simulink model "target_driver_2022_Ctrl_v_2_4_landing_2017a"  (R2017a)
settings: Solver=FixedStepDiscrete  StartTime=0.0  StopTime=13  FixedStep=0.0001  RelTol=1e-3  EnableMultiTasking=on
values from neighbouring files (symbols this model uses):
  a2_lb = -0.25    [target_driver_setup_2022_Ctrl_V_2_4.m]    (also in target_driver_setup_2022_Ctrl_V_2_4_christian.m)
  a2_openloop = -0    (= 0)    [target_driver_setup_2022_Ctrl_V_2_4.m]    (also in target_driver_setup_2022_Ctrl_V_2_4_christian.m)
  a2_ub = 0.25    [target_driver_setup_2022_Ctrl_V_2_4.m]    (also in target_driver_setup_2022_Ctrl_V_2_4_christian.m)
  adaptive_flag = 0    [target_driver_setup_2022_Ctrl_V_2_4.m]    (also in target_driver_setup_2022_Ctrl_V_2_4_christian.m)
  adaptive_gain = [gamma_adaptive, adaptive_roll_limit, adaptive_pitch_limit, adaptive_yaw_limit, c_2_adaptive, gamma_lateral_adaptive, adaptive_x_limit, adaptive_y_limit, adaptive_z_limit, c_1_adaptive]    [target_driver_setup_2022_Ctrl_V_2_4.m]    (also in target_driver_setup_2022_Ctrl_V_2_4_christian.m)
  adaptive_lateral_flag = 0    [target_driver_setup_2022_Ctrl_V_2_4.m]    (also in target_driver_setup_2022_Ctrl_V_2_4_christian.m)
  adaptive_pitch_init = 0    [target_driver_setup_2022_Ctrl_V_2_4.m]    (also in target_driver_setup_2022_Ctrl_V_2_4_christian.m)
  adaptive_pitch_limit = 0.1/(scale^2)    (= 1e-07)    [target_driver_setup_2022_Ctrl_V_2_4.m]    (also in target_driver_setup_2022_Ctrl_V_2_4_christian.m)
  adaptive_pitch_limit_low = -adaptive_pitch_limit    (= -1e-07)    [target_driver_setup_2022_Ctrl_V_2_4.m]    (also in target_driver_setup_2022_Ctrl_V_2_4_christian.m)
  adaptive_roll_init = 0    [target_driver_setup_2022_Ctrl_V_2_4.m]    (also in target_driver_setup_2022_Ctrl_V_2_4_christian.m)
  adaptive_roll_limit = 0.3/(scale^2)    (= 3e-07)    [target_driver_setup_2022_Ctrl_V_2_4.m]    (also in target_driver_setup_2022_Ctrl_V_2_4_christian.m)
  adaptive_roll_limit_low = -adaptive_roll_limit    (= -3e-07)    [target_driver_setup_2022_Ctrl_V_2_4.m]    (also in target_driver_setup_2022_Ctrl_V_2_4_christian.m)
  adaptive_x_init = 0    [target_driver_setup_2022_Ctrl_V_2_4.m]    (also in target_driver_setup_2022_Ctrl_V_2_4_christian.m)
  adaptive_x_limit = 0.15/(scale)    (= 0.00015)    [target_driver_setup_2022_Ctrl_V_2_4.m]    (also in target_driver_setup_2022_Ctrl_V_2_4_christian.m)
  adaptive_x_limit_low = -adaptive_x_limit    (= -0.00015)    [target_driver_setup_2022_Ctrl_V_2_4.m]    (also in target_driver_setup_2022_Ctrl_V_2_4_christian.m)
  adaptive_y_init = 0    [target_driver_setup_2022_Ctrl_V_2_4.m]    (also in target_driver_setup_2022_Ctrl_V_2_4_christian.m)
  adaptive_y_limit = 0.15/(scale)    (= 0.00015)    [target_driver_setup_2022_Ctrl_V_2_4.m]    (also in target_driver_setup_2022_Ctrl_V_2_4_christian.m)
  adaptive_y_limit_low = -adaptive_y_limit    (= -0.00015)    [target_driver_setup_2022_Ctrl_V_2_4.m]    (also in target_driver_setup_2022_Ctrl_V_2_4_christian.m)
  adaptive_yaw_init = 0    [target_driver_setup_2022_Ctrl_V_2_4.m]    (also in target_driver_setup_2022_Ctrl_V_2_4_christian.m)
  adaptive_yaw_limit = 0.035/(scale^2)    (= 3.5e-08)    [target_driver_setup_2022_Ctrl_V_2_4.m]    (also in target_driver_setup_2022_Ctrl_V_2_4_christian.m)
  adaptive_yaw_limit_low = -adaptive_yaw_limit    (= -3.5e-08)    [target_driver_setup_2022_Ctrl_V_2_4.m]    (also in target_driver_setup_2022_Ctrl_V_2_4_christian.m)
  adaptive_z_init = 0/scale    (= 0)    [target_driver_setup_2022_Ctrl_V_2_4.m]    (also in target_driver_setup_2022_Ctrl_V_2_4_christian.m)
  adaptive_z_limit = 0.20/(scale)    (= 0.0002)    [target_driver_setup_2022_Ctrl_V_2_4.m]    (also in target_driver_setup_2022_Ctrl_V_2_4_christian.m)
  adaptive_z_limit_low = -adaptive_z_limit/1    (= -0.0002)    [target_driver_setup_2022_Ctrl_V_2_4.m]    (also in target_driver_setup_2022_Ctrl_V_2_4_christian.m)
  att_s = 500    [target_driver_setup_2022_Ctrl_V_2_4.m]    (also in target_driver_setup_2022_Ctrl_V_2_4_christian.m)
  b_1_d_desired = [1,0,0]    [target_driver_setup_2022_Ctrl_V_2_4.m]    (also in target_driver_setup_2022_Ctrl_V_2_4_christian.m)
  closedloop_flag = 1    [target_driver_setup_2022_Ctrl_V_2_4.m]    (also in target_driver_setup_2022_Ctrl_V_2_4_christian.m)
  control_gain = [k_x,k_v, k_R, k_Omega, k_z, k_vz, k_Rx]    [target_driver_setup_2022_Ctrl_V_2_4.m]    (also in target_driver_setup_2022_Ctrl_V_2_4_christian.m)
  delay = delay-vicon_sample_cycle/2    [target_driver_setup_2022_Ctrl_V_2_4.m]    (also in target_driver_setup_2022_Ctrl_V_2_4_christian.m)
  drv_amp = 160    [target_driver_setup_2022_Ctrl_V_2_4.m]    (also in target_driver_setup_2022_Ctrl_V_2_4_christian.m)
  drv_bias = max_drv_bias    (= 300)    [target_driver_setup_2022_Ctrl_V_2_4.m]    (also in target_driver_setup_2022_Ctrl_V_2_4_christian.m)
  drv_pitch_left = 0    [target_driver_setup_2022_Ctrl_V_2_4.m]    (also in target_driver_setup_2022_Ctrl_V_2_4_christian.m)
  drv_pitch_right = 0    [target_driver_setup_2022_Ctrl_V_2_4.m]    (also in target_driver_setup_2022_Ctrl_V_2_4_christian.m)
  drv_roll = -2    [target_driver_setup_2022_Ctrl_V_2_4.m]    (also in target_driver_setup_2022_Ctrl_V_2_4_christian.m = 0)
  f_fin = f    (= 155)    [target_driver_setup_2022_Ctrl_V_2_4.m]    (also in target_driver_setup_2022_Ctrl_V_2_4_christian.m)
  f_int = f    (= 155)    [target_driver_setup_2022_Ctrl_V_2_4.m]    (also in target_driver_setup_2022_Ctrl_V_2_4_christian.m)
  g = 9.8    [target_driver_setup_2022_Ctrl_V_2_4.m]    (also in target_driver_setup_2022_Ctrl_V_2_4_christian.m)
  I_moment_vec = [Ixx, Iyy, Izz]    [target_driver_setup_2022_Ctrl_V_2_4.m]    (also in target_driver_setup_2022_Ctrl_V_2_4_christian.m)
  landing_flag = 0    [target_driver_setup_2022_Ctrl_V_2_4.m]    (also in target_driver_setup_2022_Ctrl_V_2_4_christian.m)
  landing_parameter = [start_delay+T,transition_rate, rising_time, falling_time, landing_rising_time, landing_z_decrease, landing_y_decrease, landing_x_decrease]    [target_driver_setup_2022_Ctrl_V_2_4.m]    (also in target_driver_setup_2022_Ctrl_V_2_4_christian.m = [start_delay+T, transition_rate, rising_time, falling_time, )
  low_bound = -8    [target_driver_setup_2022_Ctrl_V_2_4.m]    (also in target_driver_setup_2022_Ctrl_V_2_4_christian.m = -10)
  low_bound_eR = -0.8    [target_driver_setup_2022_Ctrl_V_2_4.m]    (also in target_driver_setup_2022_Ctrl_V_2_4_christian.m)
  low_bound_vx = -0.5    [target_driver_setup_2022_Ctrl_V_2_4.m]    (also in target_driver_setup_2022_Ctrl_V_2_4_christian.m)
  low_bound_vy = -0.5    [target_driver_setup_2022_Ctrl_V_2_4.m]    (also in target_driver_setup_2022_Ctrl_V_2_4_christian.m)
  low_bound_vz = -0.5    [target_driver_setup_2022_Ctrl_V_2_4.m]    (also in target_driver_setup_2022_Ctrl_V_2_4_christian.m)
  low_bound_x = -0.06    [target_driver_setup_2022_Ctrl_V_2_4.m]    (also in target_driver_setup_2022_Ctrl_V_2_4_christian.m)
  low_bound_y = -0.06    [target_driver_setup_2022_Ctrl_V_2_4.m]    (also in target_driver_setup_2022_Ctrl_V_2_4_christian.m)
  low_bound_z = -0.04    [target_driver_setup_2022_Ctrl_V_2_4.m]    (also in target_driver_setup_2022_Ctrl_V_2_4_christian.m)
  m = m+payload    (= 0.000124)    [target_driver_setup_2022_Ctrl_V_2_4.m]    (also in target_driver_setup_2022_Ctrl_V_2_4_christian.m = 0.000119)
  params_vec = [params_opt.delta_1, params_opt.delta_2, params_opt.delta_3, params_opt.gamma_1, params_opt.gamma_2, params_opt.gamma_3, params_opt.eta, params_opt.nu, params_opt.mu]'    [target_driver_setup_2022_Ctrl_V_2_4.m]    (also in target_driver_setup_2022_Ctrl_V_2_4_christian.m)
  phase = 0    [target_driver_setup_2022_Ctrl_V_2_4.m]    (also in target_driver_setup_2022_Ctrl_V_2_4_christian.m)
  r_desired = [default_x, default_y,z_desired]    [target_driver_setup_2022_Ctrl_V_2_4.m]    (also in target_driver_setup_2022_Ctrl_V_2_4_christian.m)
  roll_offset_angle = 0    [target_driver_setup_2022_Ctrl_V_2_4.m]    (also in target_driver_setup_2022_Ctrl_V_2_4_christian.m)
  running_time = start_delay+total_T    (= 8.5)    [target_driver_setup_2022_Ctrl_V_2_4.m]    (also in target_driver_setup_2022_Ctrl_V_2_4_christian.m = 8.4)
  running_time_control = start_delay_control+total_T+0.0    (= 8.6)    [target_driver_setup_2022_Ctrl_V_2_4.m]    (also in target_driver_setup_2022_Ctrl_V_2_4_christian.m = 8.5)
  start_delay = 2.0    (= 2)    [target_driver_setup_2022_Ctrl_V_2_4.m]    (also in target_driver_setup_2022_Ctrl_V_2_4_christian.m)
  start_delay_control = start_delay + ramp_delay    (= 2.1)    [target_driver_setup_2022_Ctrl_V_2_4.m]    (also in target_driver_setup_2022_Ctrl_V_2_4_christian.m)
  T = 0.5    [target_driver_setup_2022_Ctrl_V_2_4.m]    (also in target_driver_setup_2022_Ctrl_V_2_4_christian.m = 0.4)
  task_flag = 0    [target_driver_setup_2022_Ctrl_V_2_4.m]    (also in target_driver_setup_2022_Ctrl_V_2_4_christian.m)
  task_parameter = [radius_ref, frequency_ref, radius_ratio, lissajous_ratio, lissajous_delta, lissajous_amplitude_ratio,z_radius_ratio]    [target_driver_setup_2022_Ctrl_V_2_4.m]    (also in target_driver_setup_2022_Ctrl_V_2_4_christian.m)
  upp_bound = 8    [target_driver_setup_2022_Ctrl_V_2_4.m]    (also in target_driver_setup_2022_Ctrl_V_2_4_christian.m = 10)
  upp_bound_eR = 0.8    [target_driver_setup_2022_Ctrl_V_2_4.m]    (also in target_driver_setup_2022_Ctrl_V_2_4_christian.m)
  upp_bound_vx = 0.5    [target_driver_setup_2022_Ctrl_V_2_4.m]    (also in target_driver_setup_2022_Ctrl_V_2_4_christian.m)
  upp_bound_vy = 0.5    [target_driver_setup_2022_Ctrl_V_2_4.m]    (also in target_driver_setup_2022_Ctrl_V_2_4_christian.m)
  upp_bound_vz = 0.5    [target_driver_setup_2022_Ctrl_V_2_4.m]    (also in target_driver_setup_2022_Ctrl_V_2_4_christian.m)
  upp_bound_x = 0.06    [target_driver_setup_2022_Ctrl_V_2_4.m]    (also in target_driver_setup_2022_Ctrl_V_2_4_christian.m)
  upp_bound_y = 0.06    [target_driver_setup_2022_Ctrl_V_2_4.m]    (also in target_driver_setup_2022_Ctrl_V_2_4_christian.m)
  upp_bound_z = 0.04    [target_driver_setup_2022_Ctrl_V_2_4.m]    (also in target_driver_setup_2022_Ctrl_V_2_4_christian.m)
undefined symbols (not defined in the file or in its folder): A, Com1, DiscIntNeverNeededParam, left_mapping, left_mapping_F_to_Phi, lp_den, lp_num, none, right_mapping, right_mapping_F_to_Phi, vlp_den, vlp_num
libraries: simulink x25, xpcnilib x2, xpcseriallib x2, xpcutilitieslib x1
(part 4 of 4)

== system target_driver_2022_Ctrl_v_2_4_landing_2017a/signal generator a1/Drive_Signal/FlattenedSine1/AveragedAmp_filtered ==
  note: To avoid having signal "jump",
      | we want SMOOTH transitions
      | in frequency (i.e., a weighted sum
      | of current freq and freq some delta t ago)
  note: time constant 0.002sec
      | for 10kHz samping
  In1 : Inport
  Discrete Transfer Fcn : DiscreteTransferFcn  Numerator=[0.05]  Denominator=[1 -.95]
  Out1 : Outport
  wires:
  In1/1 -> Discrete Transfer Fcn/1
  Discrete Transfer Fcn/1 -> Out1/1

== system target_driver_2022_Ctrl_v_2_4_landing_2017a/signal generator a1/Drive_Signal1/FlattenedSine1/Amplitude Correction ==
  y : Inport
  a2 : Inport  Port=2
  Abs : Abs
  Constant : Constant  Value=1.2
  Constant1 : Constant  Value=1.1
  Divide : Product  Inputs=*/
  Product1 : Product
  Sqrt : Sqrt  SaturateOnIntegerOverflow=on
  Subtract : Sum  Inputs=+-
  y_new : Outport
  wires:
  Constant/1 -> Subtract/1
  Subtract/1 -> Sqrt/1
  Abs/1 -> Subtract/2
  a2/1 -> Abs/1
  y/1 -> Product1/1
  Product1/1 -> y_new/1
  Divide/1 -> Product1/2
  Constant1/1 -> Divide/2
  Sqrt/1 -> Divide/1

== system target_driver_2022_Ctrl_v_2_4_landing_2017a/signal generator a1/Drive_Signal1/FlattenedSine1/AveragedAmp_filtered ==
  note: To avoid having signal "jump",
      | we want SMOOTH transitions
      | in frequency (i.e., a weighted sum
      | of current freq and freq some delta t ago)
  note: time constant 0.002sec
      | for 10kHz samping
  In1 : Inport
  Discrete Transfer Fcn : DiscreteTransferFcn  Numerator=[0.05]  Denominator=[1 -.95]
  Out1 : Outport
  wires:
  In1/1 -> Discrete Transfer Fcn/1
  Discrete Transfer Fcn/1 -> Out1/1

== system target_driver_2022_Ctrl_v_2_4_landing_2017a/signal generator a2/Drive_Signal/FlattenedSine1/Amplitude Correction ==
  y : Inport
  a2 : Inport  Port=2
  Abs : Abs
  Constant : Constant  Value=1.2
  Constant1 : Constant  Value=1.1
  Divide : Product  Inputs=*/
  Product1 : Product
  Sqrt : Sqrt  SaturateOnIntegerOverflow=on
  Subtract : Sum  Inputs=+-
  y_new : Outport
  wires:
  Constant/1 -> Subtract/1
  Subtract/1 -> Sqrt/1
  Abs/1 -> Subtract/2
  a2/1 -> Abs/1
  y/1 -> Product1/1
  Product1/1 -> y_new/1
  Divide/1 -> Product1/2
  Constant1/1 -> Divide/2
  Sqrt/1 -> Divide/1

== system target_driver_2022_Ctrl_v_2_4_landing_2017a/signal generator a2/Drive_Signal1/FlattenedSine1/Amplitude Correction ==
  y : Inport
  a2 : Inport  Port=2
  Abs : Abs
  Constant : Constant  Value=1.2
  Constant1 : Constant  Value=1.1
  Divide : Product  Inputs=*/
  Product1 : Product
  Sqrt : Sqrt  SaturateOnIntegerOverflow=on
  Subtract : Sum  Inputs=+-
  y_new : Outport
  wires:
  Constant/1 -> Subtract/1
  Subtract/1 -> Sqrt/1
  Abs/1 -> Subtract/2
  a2/1 -> Abs/1
  y/1 -> Product1/1
  Product1/1 -> y_new/1
  Divide/1 -> Product1/2
  Constant1/1 -> Divide/2
  Sqrt/1 -> Divide/1

== matlab function target_driver_2022_Ctrl_v_2_4_landing_2017a/Observer for averaged system/Attitude Observer/Geometric Averaging Rotation Matix/Raw quaternion ==
  data: R input; quat output
function quat = fcn(R)
Rot = zeros(3,3);
Rot = [R(1), R(2), R(3); R(4), R(5), R(6); R(7), R(8), R(9); ];
quat = rotm2quat(Rot)';

== matlab function target_driver_2022_Ctrl_v_2_4_landing_2017a/Open_Closed_loop_selection/MATLAB Function ==
  data: time input; freq output; f_int parameter; f_fin parameter; T parameter
function freq = fcn(time, f_int, f_fin, T)
%#codegen

freq = f_int;
buffer_t = 0.0; %3.0
rel_time = time-buffer_t;
if rel_time > 0
    freq = f_int + (f_fin-f_int) * (rel_time/T);
end

if freq > f_fin
    freq = f_fin;
end

== matlab function target_driver_2022_Ctrl_v_2_4_landing_2017a/Geometric Controller/Geometric Controller ==
  data: thrust_desired output; R_cur input; R_desired input; omega input; roll_torque_desired output; omega_desired input; omega_d_dot input; x_d_ddot input; e_x input; e_v input; e_R input; e_Omega input; control_gain input; I_moment_vec input; pitch_torque_desired output; m input; g input; yaw_torque_desired output; adaptive_roll input; adaptive_pitch input; adaptive_yaw input; adaptive_x input; adaptive_y input; adaptive_z input
function [thrust_desired, roll_torque_desired, pitch_torque_desired, yaw_torque_desired] = fcn(R_cur,R_desired, omega, omega_desired, omega_d_dot,x_d_ddot,e_x,e_v,e_R,e_Omega,control_gain,I_moment_vec, m, g, adaptive_roll,adaptive_pitch, adaptive_yaw, adaptive_x,adaptive_y, adaptive_z)
% 
Rot_cur = [R_cur(1), R_cur(2), R_cur(3); R_cur(4), R_cur(5), R_cur(6); R_cur(7), R_cur(8), R_cur(9)];
Rot_desired = [R_desired(1), R_desired(2), R_desired(3); R_desired(4), R_desired(5), R_desired(6); R_desired(7), R_desired(8), R_desired(9)];

k_x=control_gain(1);
k_v=control_gain(2);
k_R=control_gain(3);
k_Omega=control_gain(4);
k_z=control_gain(5);
k_vz=control_gain(6);
k_Rx=control_gain(7);

e_3 = [0,0,1]';
I_moment = zeros(3,3);
I_moment(1,1) = I_moment_vec(1);
I_moment(2,2) = I_moment_vec(2);
I_moment(3,3) = I_moment_vec(3);

w_hat=zeros(3,3);

w_hat(1,2) = -omega(3);
w_hat(2,1) = omega(3);
w_hat(1,3) = omega(2);
w_hat(3,1) = -omega(2);
w_hat(2,3) = -omega(1);
w_hat(3,2) = omega(1);

K_X = [k_x;k_x;k_z];
K_V = [k_v;k_v;k_vz];

% Different attitude gain
K_R = [k_Rx;k_R;k_R];

% Geoemtri Controller in SE(3)

M = -K_R.*e_R - k_Omega*e_Omega + w_hat*I_moment*omega - ...
                I_moment*(w_hat*Rot_cur'*Rot_desired*omega_desired - Rot_cur'*Rot_desired*omega_d_dot);

% Adaptive torques

roll_torque_desired = M(1)-adaptive_roll;
pitch_torque_desired = M(2)-adaptive_pitch;
yaw_torque_desired = M(3)/6-adaptive_yaw;

% Geometric Lateral control in SE(3)
adaptive_lateral = [adaptive_x; adaptive_y; adaptive_z];

f = (-K_X.*e_x - K_V.*e_v -adaptive_lateral + m*g*e_3 + m*x_d_ddot)'*Rot_cur*e_3;

thrust_desired = f;




if thrust_desired >= 1.6e-3
	thrust_desired= 1.6e-3;
elseif thrust_desired <=0.5e-3
	thrust_desired=0.5e-3;
end

if roll_torque_desired >= 0.5e-6
		roll_torque_desired=0.5e-6;
elseif roll_torque_desired <= -0.6e-6
		roll_torque_desired=-0.6e-6;
end

if pitch_torque_desired >= 0.2e-6
		pitch_torque_desired=0.2e-6;
elseif pitch_torque_desired <= -0.2e-6
		pitch_torque_desired=-0.2e-6;
end

% if yaw_torque_desired >= 0.2e-7
% 		pitch_torque_desired=0.2e-7;
% elseif yaw_torque_desired <= -0.2e-7
% 		yaw_torque_desired=-0.2e-7;
% end
if yaw_torque_desired >= 0.9e-7
	yaw_torque_desired = 0.9e-7;
elseif yaw_torque_desired <= -1.0e-7
	yaw_torque_desired = -1.0e-7;
end

end

== matlab function target_driver_2022_Ctrl_v_2_4_landing_2017a/Open_Closed_loop_selection/MATLAB Function4 ==
  data: openloop_control input; closedloop_control input; drv_amp_final output; closedloop_flag input; drv_pch_final_left output; drv_pch_final_right output; drv_roll_final output; a2_final output
function [drv_amp_final, drv_pch_final_left,drv_pch_final_right, drv_roll_final, a2_final] = fcn(openloop_control, closedloop_control, closedloop_flag)

if closedloop_flag==1
    drv_amp_final =closedloop_control(1);
    drv_pch_final_left =closedloop_control(2);
		drv_pch_final_right =closedloop_control(3);
    drv_roll_final=closedloop_control(4);
		a2_final=closedloop_control(5);
else
    drv_amp_final =openloop_control(1);
    drv_pch_final_left =openloop_control(2);
		drv_pch_final_right =openloop_control(3);
    drv_roll_final=openloop_control(4);
		a2_final=openloop_control(5);
		
end

== matlab function target_driver_2022_Ctrl_v_2_4_landing_2017a/Observer for averaged system/Position Observer/Averaging position & velocity  ==
  data: r_prev input; r_prev2 input; r_prev3 input; r_cur input; update input; count input; rout_prev input; rout output; vout_prev input; vout output
function [rout, vout] = fcn(r_prev,r_prev2,r_prev3,r_cur,update, count,rout_prev,vout_prev)
%#codegen

rout = zeros(3,1);
vout = zeros(3,1);
if update>0
   rout=rout_prev; 
   vout=vout_prev;
else

    % 1 cycle average
    n= 4;
    
    rout = (r_prev+r_prev2+r_prev3+r_cur)/n;
    vout = (rout-rout_prev)*10000/(count+1);
    
  
end

end

== matlab function target_driver_2022_Ctrl_v_2_4_landing_2017a/Geometric Controller/lateral adaptive/Adaptive Control ==
  data: current_adaptive_x input; current_adaptive_y input; current_adaptive_z input; der_adaptive_torque_x output; e_x input; e_v input; adaptive_gain_limit input; der_adaptive_torque_y output; der_adaptive_torque_z output
function [der_adaptive_torque_x, der_adaptive_torque_y, der_adaptive_torque_z] = fcn(current_adaptive_x,current_adaptive_y,current_adaptive_z, e_x,e_v,adaptive_gain_limit)


% Current state of adaptation
adaptive_torque_x=current_adaptive_x;
adaptive_torque_y=current_adaptive_y;
adaptive_torque_z=current_adaptive_z;

% Adaptive control parameters
gamma_lateral_adaptive = adaptive_gain_limit(6);
adaptvie_x_limit = adaptive_gain_limit(7);
adaptvie_y_limit = adaptive_gain_limit(8);
adaptvie_z_limit = adaptive_gain_limit(9);
c_1 = adaptive_gain_limit(10);

% Flag indicating the limit
adaptive_flag_x = adaptive_torque_x*(e_v(1)+c_1*e_x(1));
adaptive_flag_y = adaptive_torque_y*(e_v(2)+c_1*e_x(2));
adaptive_flag_z = adaptive_torque_z*(e_v(3)+c_1*e_x(3));

% size(adaptive_flag_x)

% derivative for desired adaptation
der_adaptive = gamma_lateral_adaptive*(e_v+c_1*e_x);

% epsillon=1e-15;


if (adaptive_flag_x<=0 && abs(adaptive_torque_x)==adaptvie_x_limit) || abs(adaptive_torque_x)<adaptvie_x_limit
	
	der_adaptive_torque_x=der_adaptive(1);
else
	der_adaptive_torque_x = 0;
end

if (adaptive_flag_y<=0 && abs(adaptive_torque_y)==adaptvie_y_limit) || abs(adaptive_torque_y)<adaptvie_y_limit
	
	der_adaptive_torque_y=der_adaptive(2);
else
	der_adaptive_torque_y = 0;
	
end

if (adaptive_flag_z<=0 && abs(adaptive_torque_z)==adaptvie_z_limit)|| abs(adaptive_torque_z)<adaptvie_z_limit
	
	der_adaptive_torque_z=der_adaptive(3);
else
	der_adaptive_torque_z = 0;
	
end


end

== matlab function target_driver_2022_Ctrl_v_2_4_landing_2017a/Observer for averaged system/Euler derivative & filtered angular velocity /Angular velocity ==
  data: R input; Rdot input; w output; Frob_error output
function [w,Frob_error] = fcn(R,Rdot)
%#codegen
Rot = [R(1), R(2), R(3); R(4), R(5), R(6); R(7), R(8), R(9); ];
dRot = [Rdot(1), Rdot(2), Rdot(3); Rdot(4), Rdot(5), Rdot(6); Rdot(7), Rdot(8), Rdot(9); ];

A = Rot'*dRot;
w_hat = 1/2*(A-A');
w=zeros(3,1);
w(1) = w_hat(3,2);
w(2) = w_hat(1,3);
w(3) = w_hat(2,1);
% wz = w(3);
Frob_error=trace((A+A')*(A+A'));

== matlab function target_driver_2022_Ctrl_v_2_4_landing_2017a/Vicon Post Processing/Vicon Validity check/MATLAB Function3 ==
  data: R_prev input; y output; R_cur input
function y = fcn(R_prev,R_cur)
Rot_cur = [R_cur(1), R_cur(2), R_cur(3); R_cur(4), R_cur(5), R_cur(6); R_cur(7), R_cur(8), R_cur(9)];
Rot_prev = [R_prev(1), R_prev(2), R_prev(3); R_prev(4), R_prev(5), R_prev(6); R_prev(7), R_prev(8), R_prev(9)];

A=Rot_cur'*Rot_prev;
epsilonn = 1e-18;

if trace((A-eye(3))'*(A-eye(3)))<epsilonn
   y=0; 
else
    y=1;
end

== matlab function target_driver_2022_Ctrl_v_2_4_landing_2017a/Vicon correction ==
  data: x_cur input; x_corrected_vec output; roll_offset_angle input
function x_corrected_vec = fcn(x_cur,roll_offset_angle)

x_cur_vec = [x_cur(1); x_cur(2); x_cur(3)];
Rot_correction = [1, 0, 0; ...
									0, cos(roll_offset_angle), -sin(roll_offset_angle);...
									0, sin(roll_offset_angle), cos(roll_offset_angle)];
x_corrected_vec = Rot_correction*x_cur_vec;

end

== matlab function target_driver_2022_Ctrl_v_2_4_landing_2017a/Desired attitude and normalized error/saturated normalized error observation/Saturated angular velocity eOmega /Compute attitude error eR ==
  data: y output; R_cur input; R_desired input; omega input; omega_desired input
function y  = fcn(R_cur,R_desired,omega, omega_desired)

Rot_cur = [R_cur(1), R_cur(2), R_cur(3); R_cur(4), R_cur(5), R_cur(6); R_cur(7), R_cur(8), R_cur(9)];
Rot_desired = [R_desired(1), R_desired(2), R_desired(3); R_desired(4), R_desired(5), R_desired(6); R_desired(7), R_desired(8), R_desired(9)];
eOmega=zeros(3,1);
eOmega = omega - Rot_cur'*Rot_desired*omega_desired;

y = eOmega;

end

== matlab function target_driver_2022_Ctrl_v_2_4_landing_2017a/Observer for averaged system/Attitude Observer/Geometric Averaging Rotation Matix/Geometric Averaging Rotation M/Geometric Average  ==
  data: R_prev input; R_prev2 input; R_prev3 input; R_prev4 input; R_prev5 input; R_prev6 input; Rout output; R_cur input; update input; Rout_prev input
function Rout = fcn(R_prev,R_prev2,R_prev3,R_prev4,R_prev5,R_prev6,R_cur,update,Rout_prev)
%#codegen
Rot_cur = [R_cur(1), R_cur(2), R_cur(3); R_cur(4), R_cur(5), R_cur(6); R_cur(7), R_cur(8), R_cur(9)];
Rot_prev = [R_prev(1), R_prev(2), R_prev(3); R_prev(4), R_prev(5), R_prev(6); R_prev(7), R_prev(8), R_prev(9)];
Rot_prev2 = [R_prev2(1), R_prev2(2), R_prev2(3); R_prev2(4), R_prev2(5), R_prev2(6); R_prev2(7), R_prev2(8), R_prev2(9)];
Rot_prev3 = [R_prev3(1), R_prev3(2), R_prev3(3); R_prev3(4), R_prev3(5), R_prev3(6); R_prev3(7), R_prev3(8), R_prev3(9)];
Rot_prev4 = [R_prev4(1), R_prev4(2), R_prev4(3); R_prev4(4), R_prev4(5), R_prev4(6); R_prev4(7), R_prev4(8), R_prev4(9)];
Rot_prev5 = [R_prev5(1), R_prev5(2), R_prev5(3); R_prev5(4), R_prev5(5), R_prev5(6); R_prev5(7), R_prev5(8), R_prev5(9)];
Rot_prev6 = [R_prev6(1), R_prev6(2), R_prev6(3); R_prev6(4), R_prev6(5), R_prev6(6); R_prev6(7), R_prev6(8), R_prev6(9)];

Rout = zeros(9,1);
if update>0
   Rout=Rout_prev; 
else
% % 1 cycle average
%     n= 3;
%     
%     w_R0 = exp_map(Rot_cur);
%     w_R1 = exp_map(Rot_prev);
%     w_R2 = exp_map(Rot_prev2);
%     
%     
%     if sign(w_R2'*w_R0)<0
%         w_R0=-w_R0;
%     end
%     if sign(w_R2'*w_R1)<0
%         w_R1=-w_R1;
%     end
%    
%     
%     meanR0=frac_rot(w_R0,n);
%     meanR1=frac_rot(w_R1,n);
%     meanR2=frac_rot(w_R2,n);
%    
%     mean_R = meanR2*meanR1*meanR0;

% 1 cycle average
    n= 4;
    
    w_R0 = exp_map(Rot_cur);
    w_R1 = exp_map(Rot_prev);
    w_R2 = exp_map(Rot_prev2);
    w_R3 = exp_map(Rot_prev3);
    
    
    if sign(w_R3'*w_R0)<0
        w_R0=-w_R0;
    end
    if sign(w_R3'*w_R1)<0
        w_R1=-w_R1;
    end
    if sign(w_R3'*w_R2)<0
        w_R2=-w_R2;
    end
    
    meanR0=frac_rot(w_R0,n);
    meanR1=frac_rot(w_R1,n);
    meanR2=frac_rot(w_R2,n);
    meanR3=frac_rot(w_R3,n);

    mean_R = meanR3*meanR2*meanR1*meanR0;

% % 2 cycle average
%     n=7;
%     w_R0 = exp_map(Rot_cur);
%     w_R1 = exp_map(Rot_prev);
%     w_R2 = exp_map(Rot_prev2);
%     w_R3 = exp_map(Rot_prev3);
%     w_R4 = exp_map(Rot_prev4);
%     w_R5 = exp_map(Rot_prev5);
%     w_R6 = exp_map(Rot_prev6);
%     
%     if sign(w_R6'*w_R0)<0
%         w_R0=-w_R0;
%     end
%     if sign(w_R6'*w_R1)<0
%         w_R1=-w_R1;
%     end
%     if sign(w_R6'*w_R2)<0
%         w_R2=-w_R2;
%     end
%     if sign(w_R6'*w_R3)<0
%         w_R3=-w_R3;
%     end
%     if sign(w_R6'*w_R4)<0
%         w_R4=-w_R4;
%     end
%     if sign(w_R5'*w_R5)<0
%         w_R5=-w_R5;
%     end
%     meanR0=frac_rot(w_R0,n); 
%     meanR1=frac_rot(w_R1,n);
%     meanR2=frac_rot(w_R2,n);
%     meanR3=frac_rot(w_R3,n);
%     meanR4=frac_rot(w_R4,n);
%     meanR5=frac_rot(w_R5,n);
%     meanR6=frac_rot(w_R6,n);
% 
% %     mean_R = meanR3*meanR2*meanR1*meanR0;
%     mean_R = meanR6*meanR5*meanR4*meanR3*meanR2*meanR1*meanR0;
    
    Rout = [mean_R(1,1); mean_R(1,2); mean_R(1,3); mean_R(2,1); mean_R(2,2); mean_R(2,3); mean_R(3,1); mean_R(3,2); mean_R(3,3)]; 
end

end

function w = exp_map(R)

tr_R_diff = trace(R);
% isreal(tr_R_diff)
if abs((tr_R_diff-1)/2)<=1
    theta = acos((tr_R_diff-1)/2);
else
    theta=acos((tr_R_diff-1)/2/abs((tr_R_diff-1)/2));
end
if theta==0
    w= [0;0;0];
else
    w = theta/(2*sin(theta))*[R(3,2)-R(2,3); R(1,3) - R(3,1); R(2,1)-R(1,2)];
end
end

function fractional_rot = frac_rot(w,n)

w_hat = zeros(3,3);
w_hat = [0,-w(3),w(2);...
          w(3),0,-w(1);...
          -w(2), w(1), 0]/n;
fractional_rot = expm(w_hat);
end
% mean_R = R_prev_prev^(1/3)*R_prev^(1/3)*R_cur^(1/3);

% R is 1x9

== matlab function target_driver_2022_Ctrl_v_2_4_landing_2017a/Observer for averaged system/Attitude Observer/Geometric Averaging Rotation Matix/Averaged quaternion ==
  data: R input; quat output
function quat = fcn(R)
Rot = zeros(3,3);
Rot = [R(1), R(2), R(3); R(4), R(5), R(6); R(7), R(8), R(9); ];
quat = rotm2quat(Rot)';

== matlab function target_driver_2022_Ctrl_v_2_4_landing_2017a/Observer for averaged system/Attitude Observer/Geometric derivative in SO(3)/First order geometric derivative in SO(3)  ==
  data: R_prev input; omega output; R_cur input; omega_prev input; update input; count input
function omega  = fcn(R_prev, R_cur, omega_prev, update, count)

Rot_cur = [R_cur(1), R_cur(2), R_cur(3); R_cur(4), R_cur(5), R_cur(6); R_cur(7), R_cur(8), R_cur(9)];
Rot_prev = [R_prev(1), R_prev(2), R_prev(3); R_prev(4), R_prev(5), R_prev(6); R_prev(7), R_prev(8), R_prev(9)];

R_diff = Rot_prev'*Rot_cur;

tr_R_diff = trace(R_diff);
omega = zeros(3,1);
if update>0
   omega=omega_prev; 
else
    
% isreal(tr_R_diff)
if abs((tr_R_diff-1)/2)<=1
    theta = acos((tr_R_diff-1)/2);
else
    theta=acos((tr_R_diff-1)/2/abs((tr_R_diff-1)/2));
end

% To avoid NaN for omega
if theta<1e-10
	omega = omega_prev;
else
	w = 1/(2*sin(theta))*[R_diff(3,2)-R_diff(2,3); R_diff(1,3) - R_diff(3,1); R_diff(2,1)-R_diff(1,2)];

	omega = w*theta*10000/(count+1);
end   

end
% 
% if theta==0 %update~=0 
%     y = y_prev;
% else
%      w = 1/(2*sin(theta))*[R_diff(3,2)-R_diff(2,3); R_diff(1,3) - R_diff(3,1); R_diff(2,1)-R_diff(1,2)];
%      y = w*theta*10000/20;
% end

== matlab function target_driver_2022_Ctrl_v_2_4_landing_2017a/Phantom1/start at three ==
  data: time input; trigger output
function trigger = fcn(time)
%#codegen
trigger = 0;
if time > 0
   trigger = 1; 
end
if time > 0.1
   trigger = 0; 
end

== matlab function target_driver_2022_Ctrl_v_2_4_landing_2017a/Desired attitude and normalized error/saturated normalized error observation/Saturated normalized eR/Compute attitude error eR ==
  data: y output; R_cur input; R_desired input
function y  = fcn(R_cur,R_desired)

Rot_cur = [R_cur(1), R_cur(2), R_cur(3); R_cur(4), R_cur(5), R_cur(6); R_cur(7), R_cur(8), R_cur(9)];
Rot_desired = [R_desired(1), R_desired(2), R_desired(3); R_desired(4), R_desired(5), R_desired(6); R_desired(7), R_desired(8), R_desired(9)];
eR_so3=zeros(3,3);
eR_so3 = 1/2*(Rot_desired.'*Rot_cur-Rot_cur.'*Rot_desired);

eR = zeros(3,1);
eR(1) = eR_so3(3,2);
eR(2) = eR_so3(1,3);
eR(3) = eR_so3(2,1);

y = eR;

end

== matlab function target_driver_2022_Ctrl_v_2_4_landing_2017a/Force_to_Voltage1/Desired_Force_to_Voltage ==
  data: Thrust_desired input; drv_amp output; Roll_torque_desired input; Pitch_torque_desired input; Yaw_torque_desired input; drv_roll output; drv_pitch_left output; drv_pitch_right output; a2_coeff output; params_vec input
function [drv_amp, drv_roll, drv_pitch_left, drv_pitch_right, a2_coeff] =    fcn(Thrust_desired, Roll_torque_desired, Pitch_torque_desired, Yaw_torque_desired, params_vec)

% global params_opt

delta_1 = params_vec(1);
delta_2 = params_vec(2);
delta_3 = params_vec(3);
gamma_1 = params_vec(4);
gamma_2 = params_vec(5);
gamma_3 = params_vec(6);
eta = params_vec(7);
nu = params_vec(8);
mu = params_vec(9);


% Initializing for averaging filter at the end to prevent InF
if Thrust_desired==0    
    u4 = 0;
else
    u4 = Pitch_torque_desired/(Thrust_desired*delta_3*gamma_2)-nu;
end


% u3 calculation when tau approaches to zero
if abs(Yaw_torque_desired)<1e-12
    
   u3 = -mu;
else
    % Bounds for the mapping to produce real solution
    lb =(Thrust_desired/2)*(gamma_2*gamma_3*delta_2*mu/delta_1-sqrt((gamma_2*gamma_3*delta_2*Thrust_desired*mu/delta_1)^2+gamma_2*gamma_3));
    ub =(Thrust_desired/2)*(gamma_2*gamma_3*delta_2*mu/delta_1+sqrt((gamma_2*gamma_3*delta_2*Thrust_desired*mu/delta_1)^2+gamma_2*gamma_3));
   
   if Yaw_torque_desired>=ub
       Yaw_torque_desired = ub;
   elseif Yaw_torque_desired<=lb
       Yaw_torque_desired = lb; 
   end
       
   u3 = delta_1*(gamma_2*gamma_3*Thrust_desired-sqrt((gamma_2*gamma_3*Thrust_desired)^2-4*Yaw_torque_desired*(Yaw_torque_desired-gamma_2*gamma_3*delta_2*Thrust_desired*mu/delta_1)))/(2*delta_2*Yaw_torque_desired);

end

D = delta_1^2+delta_2^2*u3^2;
u1 = (gamma_2*Thrust_desired+Roll_torque_desired)/(2*gamma_1*gamma_2*D*eta);
u2 = (gamma_2*Thrust_desired-Roll_torque_desired)/(2*gamma_1*gamma_2*D);

vleft_p2p = sqrt(u1)*2;
vright_p2p = sqrt(u2)*2;
vleft_pitch = u4;
vright_pitch = u4;


drv_amp = abs((vleft_p2p-vright_p2p))/2+min(vleft_p2p,vright_p2p); % p2p
drv_roll = (vleft_p2p-vright_p2p)/4; % Amplitude
drv_pitch_left = vleft_pitch;
drv_pitch_right = vright_pitch;
a2_coeff = u3;

end

== matlab function target_driver_2022_Ctrl_v_2_4_landing_2017a/Desired attitude and normalized error/Desired_Attitude  ==
  data: R_cur input; R_d_prev input; R_d_vec output; e_x input; e_v input; x_d_ddot input; b_1_d input; control_gain input; m input; g input; update input; adaptive_lateral_control input
function R_d_vec = fcn(R_cur,R_d_prev, e_x,e_v,x_d_ddot, b_1_d, control_gain, m, g, update, adaptive_lateral_control)

R_d_vec = zeros(9,1);
data = 0;
if update>0
   R_d_vec=R_d_prev; 
	 
else
    
    k_x = control_gain(1);
    k_v = control_gain(2);
		k_z = control_gain(5);
		k_vz = control_gain(6);
		
		K_X = [k_x;k_x;k_z];
		K_V = [k_v;k_v;k_vz];

    e_3 = [0 0 1]';
%     e_1 = [1 0 0]';
		
    Rot_cur = [R_cur(1), R_cur(2), R_cur(3); R_cur(4), R_cur(5), R_cur(6); R_cur(7), R_cur(8), R_cur(9)];
		
% 		% Current heading control
%     b_1_d = Rot_cur*e_1;
% 		
% 		% Desired constant heading 
% 		b_1_d = [0 1 0]'; % e_1;
		
% Heading selection
    b_1_d = b_1_d/norm(b_1_d);

% Adaptive lateral control direction
adaptive_lateral = [adaptive_lateral_control(1); adaptive_lateral_control(2); adaptive_lateral_control(3)];
		

    b_3_d = (-K_X.*e_x - K_V.*e_v -adaptive_lateral + m*g*e_3 + m*x_d_ddot) / ...
            norm(-K_X.*e_x - K_V.*e_v -adaptive_lateral + m*g*e_3 + m*x_d_ddot);
    b_2_d = cross(b_3_d,b_1_d) / norm(cross(b_3_d,b_1_d));
		
% 		data = norm(b_2_d);
		
    % Desired rotation matrix
    R_d = [cross(b_2_d,b_3_d) b_2_d b_3_d];

    R_d_vec = [R_d(1,1); R_d(1,2); R_d(1,3); R_d(2,1); R_d(2,2); R_d(2,3); R_d(3,1); R_d(3,2); R_d(3,3)];

end



end

== matlab function target_driver_2022_Ctrl_v_2_4_landing_2017a/Force_to_Voltage1/Force to Trajectory  ==
  data: Thrust_desired input; Phi_left_p2p_desired output; Roll_torque_desired input; Pitch_torque_desired input; left_mapping_F_to_Phi input; right_mapping_F_to_Phi input; A input; Phi_right_p2p_desired output; Phi_pitch_desired output
function [Phi_left_p2p_desired, Phi_right_p2p_desired, Phi_pitch_desired] = fcn(Thrust_desired, Roll_torque_desired, Pitch_torque_desired, left_mapping_F_to_Phi, right_mapping_F_to_Phi, A)

delta_opt_L = left_mapping_F_to_Phi(1);
gamma_opt_L = left_mapping_F_to_Phi(2);
phi_opt_L = left_mapping_F_to_Phi(3);
phi_opt_offset_L = left_mapping_F_to_Phi(4);

delta_opt_R = right_mapping_F_to_Phi(1);
gamma_opt_R = right_mapping_F_to_Phi(2);
phi_opt_R = right_mapping_F_to_Phi(3);
phi_opt_offset_R = right_mapping_F_to_Phi(4);

T_thrust_roll = A*[ delta_opt_L              ,               delta_opt_R;...
                    delta_opt_L*gamma_opt_L  , - delta_opt_R*gamma_opt_R];
T_pitch_thrust = A*[delta_opt_L*gamma_opt_L  , delta_opt_R*gamma_opt_R].*[phi_opt_L, phi_opt_R];
T_pitch_offset = A*[delta_opt_L*gamma_opt_L  , delta_opt_R*gamma_opt_R].*[phi_opt_offset_L, phi_opt_offset_R];

Thrust_roll = [Thrust_desired; Roll_torque_desired];
u1_u2_desired = (T_thrust_roll)\Thrust_roll;

if (T_pitch_thrust*u1_u2_desired)==0
	Phi_pitch_desired = 0;
else
	Phi_pitch_desired = (Pitch_torque_desired-T_pitch_offset*u1_u2_desired)/(T_pitch_thrust*u1_u2_desired);
end

Phi_left_p2p_desired = sqrt(u1_u2_desired(1));
Phi_right_p2p_desired = sqrt(u1_u2_desired(2));

== matlab function target_driver_2022_Ctrl_v_2_4_landing_2017a/Desired attitude and normalized error/Geometric derivative for Rd in SO(3)/First order geometric derivative in SO(3)  ==
  data: R_prev input; omega_d output; R_cur input; omega_d_prev input; update input; count input
function omega_d   = fcn(R_prev, R_cur, omega_d_prev, update, count)

Rot_cur = [R_cur(1), R_cur(2), R_cur(3); R_cur(4), R_cur(5), R_cur(6); R_cur(7), R_cur(8), R_cur(9)];
Rot_prev = [R_prev(1), R_prev(2), R_prev(3); R_prev(4), R_prev(5), R_prev(6); R_prev(7), R_prev(8), R_prev(9)];

R_diff = Rot_prev'*Rot_cur;

tr_R_diff = trace(R_diff);
omega_d = zeros(3,1);
% omega_d_dot = zeros(3,1);

if update>0
   omega_d=omega_d_prev; 
%    omega_d_dot = omega_d_dot_prev;
else
    
% isreal(tr_R_diff)
if abs((tr_R_diff-1)/2)<=1
    theta = acos((tr_R_diff-1)/2);
else
    theta=acos((tr_R_diff-1)/2/abs((tr_R_diff-1)/2));
end

if theta==0
	theta=1e-14;
end

   w = 1/(2*sin(theta))*[R_diff(3,2)-R_diff(2,3); R_diff(1,3) - R_diff(3,1); R_diff(2,1)-R_diff(1,2)];
   omega_d = w*theta*10000/(count+1);
%    omega_d_dot = (omega_d - omega_d_prev)*10000/(count+1);
     
end
% 
% if theta==0 %update~=0 
%     y = y_prev;
% else
%      w = 1/(2*sin(theta))*[R_diff(3,2)-R_diff(2,3); R_diff(1,3) - R_diff(3,1); R_diff(2,1)-R_diff(1,2)];
%      y = w*theta*10000/20;
% end

== matlab function target_driver_2022_Ctrl_v_2_4_landing_2017a/Force_to_Voltage1/Trajectory to Voltage Input  ==
  data: Phi_left_p2p_command input; drv_amp output; Phi_right_p2p_command input; Phi_pitch_command input; drv_roll output; drv_pitch_left output; left_mapping input; right_mapping input; drv_pitch_right output
function [drv_amp, drv_roll, drv_pitch_left, drv_pitch_right] = fcn(Phi_left_p2p_command,Phi_right_p2p_command,Phi_pitch_command,left_mapping,right_mapping)

% Mapping for Voltage peak to peak from desired Stroke peak to peak
p1_left = left_mapping(1); % V_left_p2p = p1_left*Phi_p2p + p2_left
p2_left = left_mapping(2);
p1_right = right_mapping(1); % V_right_p2p = p1_right*Phi_p2p + p2_right
p2_right = right_mapping(2);

% Mapping for Voltage offset to peak from desired Stroke peak to peak
p1_pitch_left = left_mapping(3); % vleft_pitch = p1_pitch_left*Phi_pitch_command + p2_pitch_left
p2_pitch_left = left_mapping(4);
p1_pitch_right = right_mapping(3); % vright_pitch = p1_pitch_right*Phi_pitch_command + p2_pitch_right
p2_pitch_right = right_mapping(4);

vleft_p2p = p1_left*Phi_left_p2p_command + p2_left;
vright_p2p = p1_right*Phi_right_p2p_command + p2_right;
vleft_pitch = p1_pitch_left*Phi_pitch_command + p2_pitch_left;
vright_pitch = p1_pitch_right*Phi_pitch_command + p2_pitch_right;



drv_amp = abs((vleft_p2p-vright_p2p))/2+min(vleft_p2p,vright_p2p); % p2p
drv_roll = (vleft_p2p-vright_p2p)/4; % Amplitude
drv_pitch_left = vleft_pitch;
drv_pitch_right = vright_pitch;

== matlab function target_driver_2022_Ctrl_v_2_4_landing_2017a/Geometric Controller/Attitude Adaptive/Adaptive Control ==
  data: current_adaptive_roll input; current_adaptive_pitch input; current_adaptive_yaw input; der_adaptive_torque_roll output; e_R input; e_Omega input; adaptive_gain_limit input; der_adaptive_torque_pitch output; der_adaptive_torque_yaw output
function [der_adaptive_torque_roll, der_adaptive_torque_pitch, der_adaptive_torque_yaw] = fcn(current_adaptive_roll,current_adaptive_pitch,current_adaptive_yaw, e_R,e_Omega,adaptive_gain_limit)


% Current state of adaptation
adaptive_torque_roll=current_adaptive_roll;
adaptive_torque_pitch=current_adaptive_pitch;
adaptive_torque_yaw=current_adaptive_yaw;

% Adaptive control parameters
gamma_adaptive = adaptive_gain_limit(1);
adaptvie_roll_limit = adaptive_gain_limit(2);
adaptvie_pitch_limit = adaptive_gain_limit(3);
adaptvie_yaw_limit = adaptive_gain_limit(4);
c_2 = adaptive_gain_limit(5);

% Flag indicating the limit
adaptive_flag_roll = adaptive_torque_roll*(e_Omega(1)+c_2*e_R(1));
adaptive_flag_pitch = adaptive_torque_pitch*(e_Omega(2)+c_2*e_R(2));
adaptive_flag_yaw = adaptive_torque_yaw*(e_Omega(3)+c_2*e_R(3));

% size(adaptive_flag_roll)

% derivative for desired adaptation
der_adaptive = gamma_adaptive*(e_Omega+c_2*e_R);

% epsillon=1e-15;


if (adaptive_flag_roll<=0 && abs(adaptive_torque_roll)==adaptvie_roll_limit) || abs(adaptive_torque_roll)<adaptvie_roll_limit
	
	der_adaptive_torque_roll=der_adaptive(1);
else
	der_adaptive_torque_roll = 0;
end

if (adaptive_flag_pitch<=0 && abs(adaptive_torque_pitch)==adaptvie_pitch_limit) || abs(adaptive_torque_pitch)<adaptvie_pitch_limit
	
	der_adaptive_torque_pitch=der_adaptive(2);
else
	der_adaptive_torque_pitch = 0;
	
end

if (adaptive_flag_yaw<=0 && abs(adaptive_torque_yaw)==adaptvie_yaw_limit)|| abs(adaptive_torque_yaw)<adaptvie_yaw_limit
	
	der_adaptive_torque_yaw=der_adaptive(3);
else
	der_adaptive_torque_yaw = 0;
	
end


end

== matlab function target_driver_2022_Ctrl_v_2_4_landing_2017a/Vicon Post Processing/Vicon correction ==
  data: R_cur input; Rot_corrected_vec output; roll_offset_angle input
function Rot_corrected_vec = fcn(R_cur,roll_offset_angle)

Rot_cur = [R_cur(1), R_cur(2), R_cur(3); R_cur(4), R_cur(5), R_cur(6); R_cur(7), R_cur(8), R_cur(9)];
Rot_correction = [1, 0, 0; ...
									0, cos(roll_offset_angle), -sin(roll_offset_angle);...
									0, sin(roll_offset_angle), cos(roll_offset_angle)];
Rot_corrected = Rot_correction*Rot_cur;

Rot_corrected_vec = [Rot_corrected(1,1); Rot_corrected(1,2); Rot_corrected(1,3); Rot_corrected(2,1); Rot_corrected(2,2); Rot_corrected(2,3); Rot_corrected(3,1); Rot_corrected(3,2); Rot_corrected(3,3)];

end

== matlab function target_driver_2022_Ctrl_v_2_4_landing_2017a/Trajectory_generation ==
  data: task_flag input; r_desired_total output; t input; v_desired_total output; x_d_ddot_total output; b_1_d_total output; com_desired input; b_1_d_desired input; task_parameter input; landing_parameter input; landing_flag input; b_1_d_previous input
function [r_desired_total, v_desired_total, x_d_ddot_total, b_1_d_total] = fcn(task_flag, t, com_desired, b_1_d_desired, task_parameter, landing_parameter, landing_flag, b_1_d_previous)

	% 
	if task_flag == 1
		radius_ref = task_parameter(1);
		frequency_ref = task_parameter(2);
		r_desired = com_desired + radius_ref*[cos(frequency_ref*t);-sin(frequency_ref*t);0];
		v_desired = radius_ref*frequency_ref*[-sin(frequency_ref*t);-cos(frequency_ref*t);0];
		x_d_ddot  = radius_ref*frequency_ref^2*[-cos(frequency_ref*t);sin(frequency_ref*t);0];

		if radius_ref<1e-6
			b_1_d     = b_1_d_desired;
		else
			% Looking into the center
	% 		b_1_d     = (com_desired - r_desired)/norm(com_desired - r_desired);

			% Looking to the tangent

			b_1_d = v_desired/norm(v_desired);

			% Looking th camera
	% 		 b_1_d = b_1_d_desired;
		end

	elseif task_flag == 2 % Elipse
		radius_ref = task_parameter(1);
		frequency_ref = task_parameter(2);
		radius_ratio = task_parameter(3);

		r_desired = com_desired + radius_ref*[radius_ratio*cos(frequency_ref*t);-sin(frequency_ref*t);0];
		v_desired = radius_ref*frequency_ref*[-radius_ratio*sin(frequency_ref*t);-cos(frequency_ref*t);0];
		x_d_ddot  = radius_ref*frequency_ref^2*[-radius_ratio*cos(frequency_ref*t);-(-sin(frequency_ref*t));0];

		if radius_ref<1e-6
			b_1_d     = b_1_d_desired;
		else
			% Looking into the center
	% 		b_1_d     = (com_desired - r_desired)/norm(com_desired - r_desired);

			% Looking to the tangent

			b_1_d = v_desired/norm(v_desired);
		end
	elseif task_flag==3 % Vertical up and down with the landing
		radius_ref = task_parameter(1);
		frequency_ref = task_parameter(2);
		landing_time = landing_parameter(1);

		r_desired = com_desired + radius_ref*[0;0;sin(frequency_ref*(t-landing_time)-pi/2)];
		v_desired = radius_ref*frequency_ref*[0;0;cos(frequency_ref*(t-landing_time)-pi/2)];
		x_d_ddot  = radius_ref*frequency_ref^2*[0;0;-sin(frequency_ref*(t-landing_time)-pi/2)];

		if radius_ref<1e-6
			b_1_d     = b_1_d_desired;
		else
			% Looking into the center
	% 		b_1_d     = (com_desired - r_desired)/norm(com_desired - r_desired);

			% Looking to the tangent

	% 		b_1_d = v_desired/norm(v_desired);
			% Looking th camera
			 b_1_d = b_1_d_desired;
		end
	elseif task_flag==4 % circle in y-z landing
		radius_ref = task_parameter(1);
		frequency_ref = task_parameter(2);
		landing_time = landing_parameter(1);

		r_desired = com_desired + radius_ref*[0;cos(frequency_ref*(t-landing_time)-pi/2);sin(frequency_ref*(t-landing_time)-pi/2)];
		v_desired = radius_ref*frequency_ref*[0;-sin(frequency_ref*(t-landing_time)-pi/2);cos(frequency_ref*(t-landing_time)-pi/2)];
		x_d_ddot  = radius_ref*frequency_ref^2*[0;-cos(frequency_ref*(t-landing_time)-pi/2);-sin(frequency_ref*(t-landing_time)-pi/2)];

		if radius_ref<1e-6
			b_1_d     = b_1_d_desired;
		else
			% Looking into the center
	% 		b_1_d     = (com_desired - r_desired)/norm(com_desired - r_desired);

			% Looking to the tangent

	% 		b_1_d = v_desired/norm(v_desired);
			% Looking th camera
			 b_1_d = b_1_d_desired;
		end	
	elseif task_flag==5 % Lissajous curve in y-z landing
		radius_ref = task_parameter(1);
		frequency_ref = task_parameter(2);
		landing_time = landing_parameter(1);
		lissajous_ratio = task_parameter(4);
		lissajous_delta = task_parameter(5);
		lissajous_amplitude_ratio = task_parameter(6);

		r_desired = com_desired + radius_ref*[0;sin(frequency_ref*lissajous_ratio*(t-landing_time)+lissajous_delta)											;lissajous_amplitude_ratio*sin(frequency_ref*(t-landing_time))];
		v_desired = radius_ref*frequency_ref*[0;lissajous_ratio*cos(frequency_ref*lissajous_ratio*(t-landing_time)+lissajous_delta)			;lissajous_amplitude_ratio*cos(frequency_ref*(t-landing_time))];
		x_d_ddot  = radius_ref*frequency_ref^2*[0;-lissajous_ratio^2*sin(frequency_ref*lissajous_ratio*(t-landing_time)+lissajous_delta)	;-lissajous_amplitude_ratio*sin(frequency_ref*(t-landing_time))];

		if radius_ref<1e-6
			b_1_d     = b_1_d_desired;
		else

			% Looking th camera
			 b_1_d = b_1_d_desired;
		end

	elseif task_flag==6 % Elipse
		radius_ref = task_parameter(1);
		frequency_ref = task_parameter(2);
		radius_ratio = task_parameter(3);
		z_radius_ratio = task_parameter(7);

		r_desired = com_desired + radius_ref*[radius_ratio*cos(frequency_ref*t);-sin(frequency_ref*t);-z_radius_ratio*sin(frequency_ref*t)];
		v_desired = radius_ref*frequency_ref*[-radius_ratio*sin(frequency_ref*t);-cos(frequency_ref*t);-z_radius_ratio*cos(frequency_ref*t)];
		x_d_ddot  = radius_ref*frequency_ref^2*[-radius_ratio*cos(frequency_ref*t);-(-sin(frequency_ref*t));-z_radius_ratio*(-sin(frequency_ref*t))];

		if radius_ref<1e-6
			b_1_d     = b_1_d_desired;
		else
			% Looking into the center
	% 		b_1_d     = (com_desired - r_desired)/norm(com_desired - r_desired);

			% Looking to the tangent

			b_1_d = v_desired/norm(v_desired);
		end	

	elseif task_flag==7 % Elipse
		radius_ref = task_parameter(1);
		heading_vector = [0;-1;0];

		r_desired = com_desired + radius_ref*heading_vector;
		v_desired = [0;0;0];
		x_d_ddot  = [0;0;0];

		if radius_ref<1e-6
			b_1_d     = b_1_d_desired;
		else
			% Looking into the center
	% 		b_1_d     = (com_desired - r_desired)/norm(com_desired - r_desired);

			% Looking to the tangent

	% 		b_1_d = v_desired/norm(v_desired);
			% Looking at the camera
			b_1_d     = b_1_d_desired;

		end		
	elseif task_flag==8
		landing_y_decrease = landing_parameter(7);
		landing_x_decrease = landing_parameter(8);

		r_desired = com_desired+[landing_x_decrease;landing_y_decrease;0];
		v_desired = [0;0;0];
		x_d_ddot  = [0;0;0];
		b_1_d     = b_1_d_desired;

	else
		r_desired = com_desired;
		v_desired = [0;0;0];
		x_d_ddot  = [0;0;0];
		b_1_d     = b_1_d_desired;
	end

	if landing_flag==1

		trans_rate=landing_parameter(2);
		rising_time =landing_parameter(3);
		falling_time =landing_parameter(4);
		landing_rising_time = landing_parameter(5);
		landing_z_decrease = landing_parameter(6);
		landing_y_decrease = landing_parameter(7);
		landing_x_decrease = landing_parameter(8);

	% Referenece trajectory band-pass

		if task_flag==8
			rising_func = (1+tanh(trans_rate*(t-rising_time)))/2;
			fallilng_func = 0;

		else
			rising_func = (1+tanh(trans_rate*(t-rising_time)))/2-1/2;
			fallilng_func = (1-tanh(trans_rate*(t-falling_time)))/2-1/2;

		end

		landing_rising_func = (1+tanh(trans_rate*(t-landing_rising_time)))/2;

		bandpass_func = rising_func+fallilng_func;
		neg_bandpass_func = -bandpass_func+1;

		der_bandpass_func = trans_rate*(1 -(tanh(trans_rate*(t-rising_time))).^2)/2 -trans_rate*(1-(tanh(trans_rate*(t-falling_time))).^2)/2;
		dder_bandpass_func = -2*trans_rate^2*(tanh(trans_rate*(t-rising_time))).*(1 -(tanh(trans_rate*(t-rising_time))).^2)/2 +2*trans_rate^2*(tanh(trans_rate*(t-falling_time))).*(1-(tanh(trans_rate*(t-falling_time))).^2)/2;

		der_landing_func = trans_rate*(1 -(tanh(trans_rate*(t-landing_rising_time))).^2)/2;
		dder_landing_func = -2*trans_rate^2*(tanh(trans_rate*(t-landing_rising_time))).*(1 -(tanh(trans_rate*(t-landing_rising_time))).^2)/2;

		landing_desired = com_desired+[landing_x_decrease;landing_y_decrease;landing_z_decrease];
	% 	landing_desired = com_desired+[0;0;landing_z_decrease];

		if task_flag==8 % Landing only z direction at r_desired point
			r_desired_total = com_desired + bandpass_func.*(r_desired-com_desired)+landing_rising_func.*(landing_desired-r_desired);
		else
			r_desired_total = com_desired + bandpass_func.*(r_desired-com_desired)+landing_rising_func.*(landing_desired-com_desired);	
		end

		v_desired_total = der_bandpass_func.*(r_desired-com_desired) + bandpass_func.*v_desired + der_landing_func.*(landing_desired-com_desired);
		x_d_ddot_total = dder_bandpass_func.*(r_desired-com_desired) + 2*der_bandpass_func.*v_desired+ bandpass_func.*x_d_ddot+ dder_landing_func.*(landing_desired-com_desired);

	% Heading trajectory band-pass
		trans_heading_rate = trans_rate*1/1;
		rising_heading_func = (1+tanh(trans_heading_rate*(t-(rising_time+1))))/2-1/2;
		fallilng_heading_func = (1-tanh(trans_heading_rate*(t-falling_time+1)))/2-1/2;
	% rising_heading_func = (1+tanh(trans_heading_rate*(t-(rising_time))))/2-1/2;
	% 	fallilng_heading_func = (1-tanh(trans_heading_rate*(t-falling_time)))/2-1/2;


		bandpass_heading_func = rising_heading_func+fallilng_heading_func;
		neg_bandpass_heading_func = -bandpass_heading_func+1;
		landing_rising_heading_func = (1+tanh(trans_heading_rate*(t-landing_rising_time)))/2;
	% 
	% 	if norm(v_desired_total)<1e-6
	% 		b_1_d     = b_1_d_desired;
	% 	else
	% 		b_1_d = v_desired_total/norm(v_desired_total);
	% 	end
	% 	
	% 	b_1_d_total = b_1_d_desired.*neg_bandpass_heading_func + b_1_d.*bandpass_heading_func;
	% 	
	% 	b_1_d_total = b_1_d_total/norm(b_1_d_total);
	% 	
	% 		% Convex combination of the heading vector
	% 	% Linear convex comb
	% 	b_1_d_total = b_1_d_desired.*neg_bandpass_func + b_1_d.*bandpass_func;


	% Slerp for smooth heading transition
	% STEP 1 : Hovering to Desired trajectory to Hovering

		if t<rising_time && bandpass_heading_func<1e-5%1e-6
			b_1_d_current = b_1_d_desired;
		else
			b_1_d_current = b_1_d_previous;
		end


		cos_Omega_slerp = b_1_d.'*b_1_d_current;
		Omega_slerp = acos(cos_Omega_slerp);

		if Omega_slerp<1e-8
			b_1_d_total = b_1_d_current.*neg_bandpass_heading_func + b_1_d.*bandpass_heading_func;
		else
			b_1_d_total = sin(neg_bandpass_heading_func*Omega_slerp)/sin(Omega_slerp)*b_1_d_current + sin(bandpass_heading_func*Omega_slerp)/sin(Omega_slerp)*b_1_d;
		end

	% STEP 2 : Hovering to Desired Heading for landing

		b_1_d_total = sin(1-landing_rising_heading_func)*b_1_d_total + sin(landing_rising_heading_func)*b_1_d_desired;

		b_1_d_total = b_1_d_total/norm(b_1_d_total);

	else
		r_desired_total = r_desired;
		v_desired_total = v_desired;
		x_d_ddot_total = x_d_ddot;
		b_1_d_total = b_1_d;

	end
end
